simulink model "FuzzyChild"  (R2024a)
settings: Solver=FixedStepAuto  StartTime=0.0  StopTime=10.0  RelTol=1e-3
model workspace (MAT data in the model file):
  gainVal = 1
libraries: androidaudiovideolib x5, androiduilib x5, androidsensorlib x2, androidcommunicationlib x2, fuzblock x1
settings Model: Creator=srira  LastModifiedBy=Shesh
settings OptimizationCC: EnhancedBackFolding=on  PassReuseOutputArgsThreshold=0  MaxStackSize=64  OptimizeBlockOrder=speed  DifferentSizesBufferReuse=on  OptimizationCustomize=off
settings DebuggingCC: ParameterTunabilityLossMsg=error
settings HardwareCC: ProdBitPerPointer=32  ProdBitPerSizeT=32  ProdBitPerPtrDiffT=32  ProdLargestAtomicInteger=Long  ProdLargestAtomicFloat=Double  ProdWordSize=32  ProdHWDeviceType=ARM Compatible->ARM Cortex  UseEmbeddedCoderFeatures=off  UseSimulinkCoderFeatures=off
settings SFSimCC: MATLABDynamicMemAlloc=off
settings RTWCC: Description=Embedded Coder  SystemTargetFile=ert.tlc  HardwareBoard=Android Device  TLCOptions="-aInlineSetEventsForThisBaseRateFcn=TLC_FALSE -aSuppressMultiTaskScheduler=TLC_FALSE  -aRateBasedStepFcn=0"  TemplateMakefile=ert_default_tmf  RTWVerbose=off  Toolchain=Android SDK/NDK Tools  GPUComputeCapability=3.5
settings CodeAppCC: ForceParamTrailComments=on  OperatorAnnotations=on
settings ERTTargetCC: ERTCustomFileBanners=off  SupportContinuousTime=on  SupportNonInlinedSFcns=on  RemoveResetFunc=off  ModelStepFunctionPrototypeControlCompliant=off

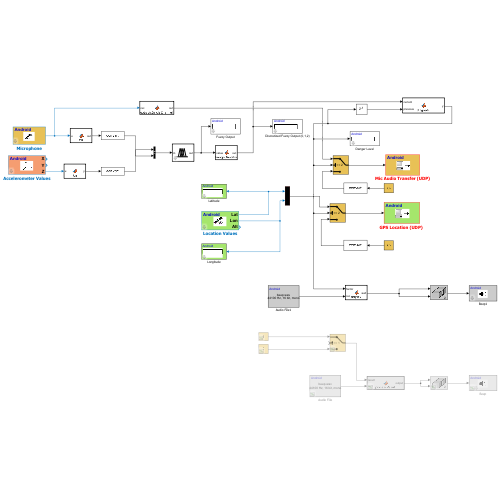
[thumbnail: Simulink's stored preview of the top-level diagram]
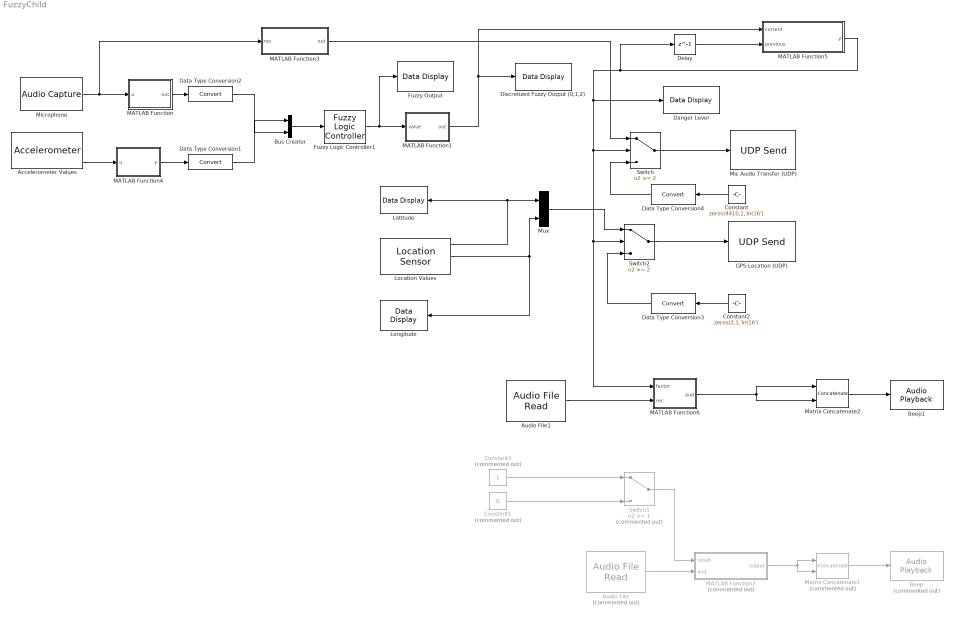
== system FuzzyChild ==
  Accelerometer Values : androidsensorlib/Accelerometer  OutputVector=off  SampleTime=0.1  BlockPlatform=Android
  Audio FIle : androidaudiovideolib/Audio File Read  Commented=on  FileName=C:\Users\Shesh\Documents\MATLAB\snake\Fall_Detection\beep.wav  FrameSize=4410
  Audio FIle1 : androidaudiovideolib/Audio File Read  FileName=C:\Users\Shesh\Documents\MATLAB\snake\Fall_Detection\beep.wav  FrameSize=4410
  Beep : androidaudiovideolib/Audio Playback  Commented=on  SampleFreq=44100  AudioSamplingFreq=44100  SampleTime=0.1  DeviceStr=0  QueueDuration=0  BlockPlatform=Android
  Beep1 : androidaudiovideolib/Audio Playback  SampleFreq=44100  AudioSamplingFreq=44100  SampleTime=0.1  DeviceStr=0  QueueDuration=0  BlockPlatform=Android
  Bus Creator : BusCreator  Inputs=2
  Constant : Constant  Value=zeros(4410,1,'int16')  VectorParams1D=off
  Constant1 : Constant  Commented=on  Value=0  VectorParams1D=off  OutDataTypeStr=Inherit: Inherit via back propagation
  Constant2 : Constant  Value=zeros(2,1,'int16')  VectorParams1D=off  OutDataTypeStr=Inherit: Inherit via back propagation
  Constant3 : Constant  Commented=on  VectorParams1D=off  OutDataTypeStr=Inherit: Inherit via back propagation
  Danger Level : androiduilib/Data Display  DataDisplayId=FuzzyChild/Danger_Level  Format=Integer  Precision=6  SimulateUsing=Code generation  blockPlatform=Android
  Data Type Conversion{1..4} (4 alike) : DataTypeConversion  SaturateOnIntegerOverflow=off  RndMeth=Floor
  Delay : Delay  DelayLength=1  InitialCondition=0
  Discretized Fuzzy Output (0,1,2) : androiduilib/Data Display  DataDisplayId=FuzzyChild/Discretized_Fuzzy_Output_(0,1,2)  Format=Integer  Precision=6  SimulateUsing=Code generation  blockPlatform=Android
  Fuzzy Logic Controller1 : fuzblock/Fuzzy Logic  Controller  FIS='Control_Systems.fis'  OutputSampleNumber=101  DataType=double  FuzzifiedInputs=off  RuleFiringStrengths=off  RuleOutputs=off  AggregatedOutputs=off  SimulateUsing=Interpreted execution  OutOfRangeInputValueMessage=warning  NoRuleFiredMessage=warning  EmptyOutputFuzzySetMessage=warning
  Fuzzy Output : androiduilib/Data Display  DataDisplayId=FuzzyChild/Fuzzy_Output  Format=Float  Precision=6  SimulateUsing=Code generation  blockPlatform=Android
  "GPS Location (UDP) " : androidcommunicationlib/UDP Send  remoteURL='10.7.31.43'  remotePort=25002  localURL='0.0.0.0'  localPortSource=Automatically determine  localPort=-1  sampletime=-1  blockPlatform=Android  separateLengthPort=0
  Latitude : androiduilib/Data Display  DataDisplayId=FuzzyChild/Latitude  Format=Float  Precision=10  SimulateUsing=Code generation  blockPlatform=Android
  Location Values : androidsensorlib/Location Sensor  OutputVector=off  SampleTime=0.1  BlockPlatform=Android
  Longitude : androiduilib/Data Display  DataDisplayId=FuzzyChild/Longitude  Format=Float  Precision=10  SimulateUsing=Code generation  blockPlatform=Android
  MATLAB Function : MATLAB Function  TreatAsAtomicUnit=on
  MATLAB Function1 : MATLAB Function  TreatAsAtomicUnit=on
  MATLAB Function2 : MATLAB Function  Commented=on  TreatAsAtomicUnit=on
  MATLAB Function3 : MATLAB Function  TreatAsAtomicUnit=on
  MATLAB Function4 : MATLAB Function  TreatAsAtomicUnit=on
  MATLAB Function5 : MATLAB Function  TreatAsAtomicUnit=on
  MATLAB Function6 : MATLAB Function  TreatAsAtomicUnit=on
  Matrix Concatenate1 : Concatenate  Commented=on  Mode=Multidimensional array  ConcatenateDimension=2
  Matrix Concatenate2 : Concatenate  Mode=Multidimensional array  ConcatenateDimension=2
  Mic Audio Transfer (UDP) : androidcommunicationlib/UDP Send  remoteURL='10.7.31.43'  remotePort=25001  localURL='0.0.0.0'  localPortSource=Automatically determine  localPort=-1  sampletime=-1  blockPlatform=Android  separateLengthPort=0
  Microphone : androidaudiovideolib/Audio Capture  SampleFreq=44100  FrameSize=4410  SampleTime=0.1  SimulateUsing=Code generation  DeviceStr=0  QueueDuration=0  BlockPlatform=Android  AudioSamplingFreq=44100
  Mux : Mux  Inputs=2
  Switch : Switch  Threshold=2  SaturateOnIntegerOverflow=off  InputSameDT=off
  Switch1 : Switch  Commented=on  Threshold=1  OutDataTypeStr=Inherit: Inherit via back propagation  SaturateOnIntegerOverflow=off  InputSameDT=off
  Switch2 : Switch  Threshold=2  OutDataTypeStr=Inherit: Inherit via back propagation  SaturateOnIntegerOverflow=off  InputSameDT=off
  wires:
  Constant/1 -> Data Type Conversion4/1
  Constant2/1 -> Data Type Conversion3/1
  Mux/1 -> Switch2/1
  Microphone/1 -> MATLAB Function/1(u), MATLAB Function3/1(rec)
  MATLAB Function2/1(output) -> Matrix Concatenate1/2, Matrix Concatenate1/1
  Matrix Concatenate1/1 -> Beep/1
  Accelerometer Values/3 -> MATLAB Function4/1(u)
  Location Values/1 -> Mux/1, Latitude/1
  Location Values/2 -> Mux/2, Longitude/1
  Audio FIle/1 -> MATLAB Function2/2(aud)
  MATLAB Function/1(out) -> Data Type Conversion2/1
  Switch/1 -> Mic Audio Transfer (UDP)/1
  Switch2/1 -> "GPS Location (UDP) "/1
  Data Type Conversion3/1 -> Switch2/3
  Data Type Conversion4/1 -> Switch/3
  Switch1/1 -> MATLAB Function2/1(result)
  Constant1/1 -> Switch1/3
  MATLAB Function1/1(out) -> MATLAB Function5/1(current), Discretized Fuzzy Output (0,1,2)/1
  Constant3/1 -> Switch1/1
  MATLAB Function4/1(y) -> Data Type Conversion1/1
  Data Type Conversion2/1 -> Bus Creator/2
  Data Type Conversion1/1 -> Bus Creator/1
  Bus Creator/1 -> Fuzzy Logic Controller1/1
  Fuzzy Logic Controller1/1 -> MATLAB Function1/1(value), Fuzzy Output/1
  MATLAB Function3/1(out) -> Switch/1
  MATLAB Function5/1(y) -> Danger Level/1, Switch/2, Switch2/2, MATLAB Function6/1(factor), Delay/1
  Delay/1 -> MATLAB Function5/2(previous)
  Matrix Concatenate2/1 -> Beep1/1
  MATLAB Function6/1(aud) -> Matrix Concatenate2/1, Matrix Concatenate2/2
  Audio FIle1/1 -> MATLAB Function6/2(rec)

== matlab function FuzzyChild/MATLAB Function ==
  data: u input; out output
 function out = fcn(u)

avg_col1 = mean(abs(u(:, 1)));
avg_col2 = mean(abs(u(:, 2)));

out = max([avg_col1, avg_col2]);

== matlab function FuzzyChild/MATLAB Function2 ==
  data: result input; output output; aud input
function output = processResult(result, aud)
    if result == 1
        output = aud;
    else
        output = zeros(4410,1,'int16');
    end
end

== matlab function FuzzyChild/MATLAB Function3 ==
  data: rec input; out output
function out = extractsSingleChannel(rec)
    out = rec(:,1);

== matlab function FuzzyChild/MATLAB Function4 ==
  data: u input; y output
function y = fcn(u)

y = abs(u);

== matlab function FuzzyChild/MATLAB Function5 ==
  data: current input; y output; previous input
function y = stagnate(current, previous)

y = max(current,previous);

== matlab function FuzzyChild/MATLAB Function6 ==
  data: factor input; aud output; rec input
function aud = amplify(factor, rec)
    aud = rec * factor^3;

== matlab function FuzzyChild/MATLAB Function1 ==
  data: value input; out output
function out = RangeClassifier(value)

  ranges = {[0, 0.38], [0.38, 0.6], [0.6, 1]};
  
  for i = 1:length(ranges)
    lower = ranges{i}(1);
    upper = ranges{i}(2);
    if (value >= lower) && (value < upper)
      out = i - 1;  % Adjust index for 0-based output (0, 1, 2)
      return;
    end
  end
  
  out = -1;
end
